simulink model "vloop"  (Simulink 7.4)
settings: Solver=ode15s  StartTime=0.0  StopTime=1  RelTol=1e-3
InitFcn:
  | G = 107.815;
libraries: simulink x1
settings Model: Creator=pic  LastModifiedBy=corkep
settings DataIOCC: LimitDataPoints=off

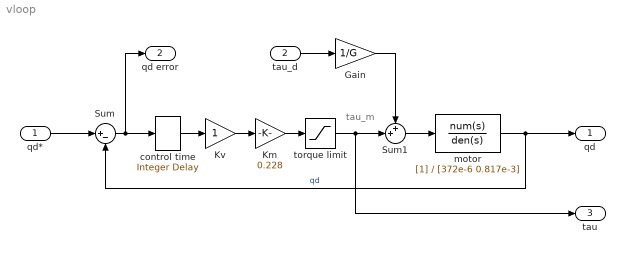
== system vloop ==
  note: tau_m
  qd* : Inport  OutDataType=fixdt(1, 16)  OutScaling=2^0
  tau_d : Inport  Port=2  OutDataType=fixdt(1, 16)  OutScaling=2^0
  Gain : Gain  Gain=1/G  ParameterDataType=fixdt(1, 16)  ParameterScaling=2^0  OutDataType=fixdt(1, 16)  OutScaling=2^0
  Km : Gain  Gain=0.228  ParameterDataType=fixdt(1, 16)  ParameterScaling=2^0  OutDataType=fixdt(1, 16)  OutScaling=2^0
  Kv : Gain  ParameterDataType=fixdt(1, 16)  ParameterScaling=2^0  OutDataType=fixdt(1, 16)  OutScaling=2^0
  Sum : Sum  Inputs=|+-  OutDataType=fixdt(1, 16)  OutScaling=2^0
  Sum1 : Sum  Inputs=++|  OutDataType=fixdt(1, 16)  OutScaling=2^0
  control time : simulink/Discrete/Integer Delay  vinit=0.0  samptime=0.001  NumDelays=1
  motor : TransferFcn  Denominator=[372e-6 0.817e-3]  ContinuousStateAttributes='qd'
  torque limit : Saturate  UpperLimit=0.9  LowerLimit=-0.9  OutDataType=fixdt(1, 16)  OutScaling=2^0
  qd : Outport  OutDataType=fixdt(1, 16)  OutScaling=2^0
  qd error : Outport  Port=2  OutDataType=fixdt(1, 16)  OutScaling=2^0
  tau : Outport  Port=3  OutDataType=fixdt(1, 16)  OutScaling=2^0
  wires:
  Gain/1 -> Sum1/1
  Sum1/1 -> motor/1
  Km/1 -> torque limit/1
  Kv/1 -> Km/1
  Sum/1 -> control time/1, qd error/1
  motor/1 -> Sum/2, qd/1  "qd"
  tau_d/1 -> Gain/1
  torque limit/1 -> Sum1/2, tau/1
  control time/1 -> Kv/1
  qd*/1 -> Sum/1
